simulink model "simu_TWIP"  (R2017a)
settings: Solver=VariableStepAuto  StartTime=0.0  StopTime=10.0  RelTol=1e-3
undefined symbols (not defined in the file or in its folder): Twip, U
settings Model: Creator=Daniel  LastModifiedBy=Daniel

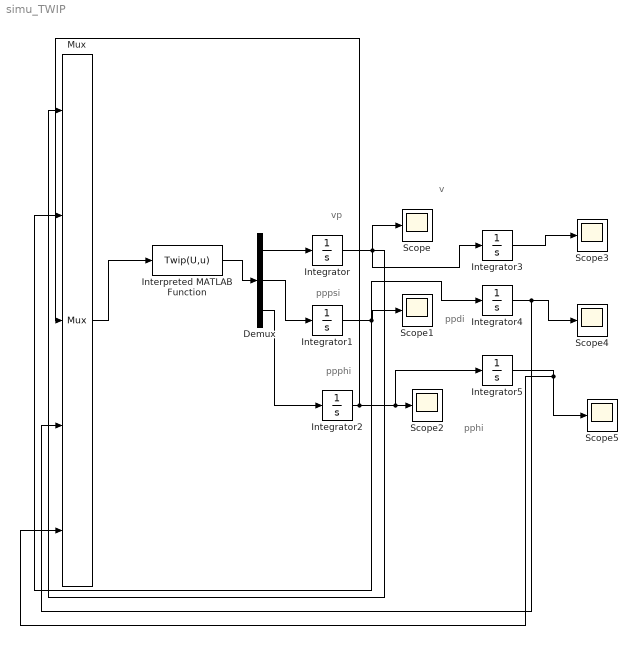
== system simu_TWIP ==
  note: pphi
  note: ppdi
  note: v
  note: ppphi
  note: pppsi
  note: vp
  Demux : Demux  Outputs=3
  Integrator{,1..5} (6 alike) : Integrator
  Interpreted MATLAB Function : MATLABFcn  MATLABFcn=Twip(U,u)
  Mux : Mux  Inputs=5
  Scope{,1..5} (6 alike) : Scope
  wires:
  Mux/1 -> Interpreted MATLAB Function/1
  Interpreted MATLAB Function/1 -> Demux/1
  Demux/1 -> Integrator/1
  Demux/2 -> Integrator1/1
  Demux/3 -> Integrator2/1
  Integrator/1 -> Mux/1, Scope/1, Integrator3/1
  Integrator1/1 -> Mux/2, Integrator4/1, Scope1/1
  Integrator2/1 -> Mux/3, Integrator5/1, Scope2/1
  Integrator3/1 -> Scope3/1
  Integrator5/1 -> Mux/5, Scope5/1
  Integrator4/1 -> Mux/4, Scope4/1
